simulink model "PannelTest"  (R2022b)
settings: Solver=FixedStepAuto  StartTime=0.0  StopTime=102  FixedStep=0.001  RelTol=1e-3
model workspace (MAT data in the model file):
  Manual_Auto : Simulink.Parameter (value not decoded)
  Pattern : Simulink.Parameter (value not decoded)
  Pause_Start : Simulink.Parameter (value not decoded)
  Stop : Simulink.Parameter (value not decoded)
  Unlock_Lock : Simulink.Parameter (value not decoded)
undefined symbols (not defined in the file or in its folder): DiscIntNeverNeededParam
(part 3 of 3)

== stateflow chart PannelTest/PanelController/ControlPannelStateMachine ==
  state Pause
    State = "Pause";
    if(Pause_StartButtonPressed==0)
    Pause_StartButtonPressed_temp = 0;
    end
  state Stop
    (history)
    state Stop
      State = "Stop";
    state LowerLimb_Follow
      state LowerLimb_Follow
        if(PatternButtonPressed==0)
        PatternButtonPressed_temp = 0;
        end
        State = "Stop";
        Mode = "Lower_Limb_Follow";
        ManualAuto = "";
      (default) -> Stop.LowerLimb_Follow.LowerLimb_Follow
    state LowerLimb_FlutterKick
      (history)
      state LowerLimb_FlutterKick
        if(PatternButtonPressed==0)
        PatternButtonPressed_temp = 0;
        end
        State = "Stop";
        Mode = "Lower_Limb_FlutterKick";
      state LLFK_Manual_Torque
        if(PatternButtonPressed==0)
        PatternButtonPressed_temp = 0;
        end
        if(Manual_AutoButtonPressed==0)
        Manual_AutoButtonPressed_temp = 0;
        end
        State = "Stop";
        Mode = "Lower_Limb_FlutterKick";
        ManualAuto = "LLFK_Manual_Torque";
      state LLFK_Manual_Freq
        if(PatternButtonPressed==0)
        PatternButtonPressed_temp = 0;
        end
        if(Manual_AutoButtonPressed==0)
        Manual_AutoButtonPressed_temp = 0;
        end
        State = "Stop";
        Mode = "Lower_Limb_FlutterKick";
        ManualAuto = "LLFK_Manual_Freq";
      state LLFK_Manual_Pos
        if(PatternButtonPressed==0)
        PatternButtonPressed_temp = 0;
        end
        if(Manual_AutoButtonPressed==0)
        Manual_AutoButtonPressed_temp = 0;
        end
        State = "Stop";
        Mode = "Lower_Limb_FlutterKick";
        ManualAuto = "LLFK_Manual_Pos";
      state LLFK_Auto
        if(PatternButtonPressed==0)
        PatternButtonPressed_temp = 0;
        end
        if(Manual_AutoButtonPressed==0)
        Manual_AutoButtonPressed_temp = 0;
        end
        State = "Stop";
        Mode = "Lower_Limb_FlutterKick";
        ManualAuto = "LLFK_Auto";
      (default) -> Stop.LowerLimb_FlutterKick.LowerLimb_FlutterKick
      Stop.LowerLimb_FlutterKick.LowerLimb_FlutterKick -> LLFK_Manual_Freq
      LLFK_Manual_Freq -> LLFK_Manual_Torque : [(Manual_AutoButtonPressed_temp==0)&&(Manual_AutoButtonPressed>0)]{Manual_AutoButtonPressed_temp=1;}
      LLFK_Manual_Torque -> LLFK_Manual_Pos : [(Manual_AutoButtonPressed_temp==0)&&(Manual_AutoButtonPressed>0)]{Manual_AutoButtonPressed_temp=1;}
      LLFK_Auto -> LLFK_Manual_Freq : [(Manual_AutoButtonPressed_temp==0)&&(Manual_AutoButtonPressed>0)]{Manual_AutoButtonPressed_temp=1;}
      LLFK_Manual_Pos -> LLFK_Auto : [(Manual_AutoButtonPressed_temp==0)&&(Manual_AutoButtonPressed>0)]{Manual_AutoButtonPressed_temp=1;}
    state LowerLimb_Breaststroke
      (history)
      state Lower_Limb_Breaststroke
        if(PatternButtonPressed==0)
        PatternButtonPressed_temp = 0;
        end
        State = "Stop";
        Mode = "Lower_Limb_Breaststroke";
      state LLB_Manual_Torque
        if(PatternButtonPressed==0)
        PatternButtonPressed_temp = 0;
        end
        if(Manual_AutoButtonPressed==0)
        Manual_AutoButtonPressed_temp = 0;
        end
        State = "Stop";
        Mode = "Lower_Limb_Breaststroke";
        ManualAuto = "LLB_Manual_Torque";
      state LLB_Manual_Freq
        if(PatternButtonPressed==0)
        PatternButtonPressed_temp = 0;
        end
        if(Manual_AutoButtonPressed==0)
        Manual_AutoButtonPressed_temp = 0;
        end
        State = "Stop";
        Mode = "Lower_Limb_Breaststroke";
        ManualAuto = "LLB_Manual_Freq";
      state LLB_Manual_Pos
        if(PatternButtonPressed==0)
        PatternButtonPressed_temp = 0;
        end
        if(Manual_AutoButtonPressed==0)
        Manual_AutoButtonPressed_temp = 0;
        end
        State = "Stop";
        Mode = "Lower_Limb_Breaststroke";
        ManualAuto = "LLB_Manual_Pos";
      state LLB_Auto
        if(PatternButtonPressed==0)
        PatternButtonPressed_temp = 0;
        end
        if(Manual_AutoButtonPressed==0)
        Manual_AutoButtonPressed_temp = 0;
        end
        State = "Stop";
        Mode = "Lower_Limb_Breaststroke";
        ManualAuto = "LLB_Auto";
      (default) -> Lower_Limb_Breaststroke
      Lower_Limb_Breaststroke -> LLB_Manual_Freq
      LLB_Manual_Freq -> LLB_Manual_Torque : [(Manual_AutoButtonPressed_temp==0)&&(Manual_AutoButtonPressed>0)]{Manual_AutoButtonPressed_temp=1;}
      LLB_Manual_Torque -> LLB_Manual_Pos : [(Manual_AutoButtonPressed_temp==0)&&(Manual_AutoButtonPressed>0)]{Manual_AutoButtonPressed_temp=1;}
      LLB_Auto -> LLB_Manual_Freq : [(Manual_AutoButtonPressed_temp==0)&&(Manual_AutoButtonPressed>0)]{Manual_AutoButtonPressed_temp=1;}
      LLB_Manual_Pos -> LLB_Auto : [(Manual_AutoButtonPressed_temp==0)&&(Manual_AutoButtonPressed>0)]{Manual_AutoButtonPressed_temp=1;}
    state LowerLimb_Walk
      (history)
      state LowerLimb_Walk
        if(PatternButtonPressed==0)
        PatternButtonPressed_temp = 0;
        end
        State = "Stop";
        Mode = "Lower_Limb_Walk";
      state LLW_Manual_Torque
        if(PatternButtonPressed==0)
        PatternButtonPressed_temp = 0;
        end
        if(Manual_AutoButtonPressed==0)
        Manual_AutoButtonPressed_temp = 0;
        end
        State = "Stop";
        Mode = "Lower_Limb_Walk";
        ManualAuto = "LLW_Manual_Torque";
      state LLW_Manual_Freq
        if(PatternButtonPressed==0)
        PatternButtonPressed_temp = 0;
        end
        if(Manual_AutoButtonPressed==0)
        Manual_AutoButtonPressed_temp = 0;
        end
        State = "Stop";
        Mode = "Lower_Limb_Walk";
        ManualAuto = "LLW_Manual_Freq";
      state LLW_Manual_Pos
        if(PatternButtonPressed==0)
        PatternButtonPressed_temp = 0;
        end
        if(Manual_AutoButtonPressed==0)
        Manual_AutoButtonPressed_temp = 0;
        end
        State = "Stop";
        Mode = "Lower_Limb_Walk";
        ManualAuto = "LLW_Manual_Pos";
      state LLW_Auto
        if(PatternButtonPressed==0)
        PatternButtonPressed_temp = 0;
        end
        if(Manual_AutoButtonPressed==0)
        Manual_AutoButtonPressed_temp = 0;
        end
        State = "Stop";
        Mode = "Lower_Limb_Walk";
        ManualAuto = "LLW_Auto";
      (default) -> Stop.LowerLimb_Walk.LowerLimb_Walk
      Stop.LowerLimb_Walk.LowerLimb_Walk -> LLW_Manual_Freq
      LLW_Manual_Freq -> LLW_Manual_Torque : [(Manual_AutoButtonPressed_temp==0)&&(Manual_AutoButtonPressed>0)]{Manual_AutoButtonPressed_temp=1;}
      LLW_Manual_Torque -> LLW_Manual_Pos : [(Manual_AutoButtonPressed_temp==0)&&(Manual_AutoButtonPressed>0)]{Manual_AutoButtonPressed_temp=1;}
      LLW_Auto -> LLW_Manual_Freq : [(Manual_AutoButtonPressed_temp==0)&&(Manual_AutoButtonPressed>0)]{Manual_AutoButtonPressed_temp=1;}
      LLW_Manual_Pos -> LLW_Auto : [(Manual_AutoButtonPressed_temp==0)&&(Manual_AutoButtonPressed>0)]{Manual_AutoButtonPressed_temp=1;}
    (default) -> Stop.Stop
    Stop.Stop -> Stop.LowerLimb_Follow
    Stop.LowerLimb_Follow -> Stop.LowerLimb_FlutterKick : [(PatternButtonPressed_temp==0)&&(PatternButtonPressed>0)]{PatternButtonPressed_temp=1;}
    LowerLimb_Breaststroke -> Stop.LowerLimb_Walk : [(PatternButtonPressed_temp==0)&&(PatternButtonPressed>0)]{PatternButtonPressed_temp=1;}
    Stop.LowerLimb_FlutterKick -> LowerLimb_Breaststroke : [(PatternButtonPressed_temp==0)&&(PatternButtonPressed>0)]{PatternButtonPressed_temp=1;}
    Stop.LowerLimb_Walk -> Stop.LowerLimb_Follow : [(PatternButtonPressed_temp==0)&&(PatternButtonPressed>0)]{PatternButtonPressed_temp=1;}
  state Start
    state Start
      State = "Start";
      if(Pause_StartButtonPressed==0)
      Pause_StartButtonPressed_temp = 0;
      end
    state UpperLimb_Lock
      if(Pause_StartButtonPressed==0)
      Pause_StartButtonPressed_temp = 0;
      end
      if(Unlock_LockButtonPressed==0)
      Unlock_LockButtonPressed_temp = 0;
      end
      State = "Start";
      UnlockLock = "UpperLimb_Lock";
    state UpperLimb_UnLock
      if(Pause_StartButtonPressed==0)
      Pause_StartButtonPressed_temp = 0;
      end
      if(Unlock_LockButtonPressed==0)
      Unlock_LockButtonPressed_temp = 0;
      end
      State = "Start";
      UnlockLock = "UpperLimb_Unlock";
    (default) -> Start.Start
    Start.Start -> UpperLimb_UnLock
    UpperLimb_Lock -> UpperLimb_UnLock : [(Unlock_LockButtonPressed_temp==0)&&(Unlock_LockButtonPressed>0)]{Unlock_LockButtonPressed_temp=1;}
    UpperLimb_UnLock -> UpperLimb_Lock : [(Unlock_LockButtonPressed_temp==0)&&(Unlock_LockButtonPressed>0)]{Unlock_LockButtonPressed_temp=1;}
  Start -> Pause : [(Pause_StartButtonPressed_temp==0)&&(Pause_StartButtonPressed>0)]{Pause_StartButtonPressed_temp=1;UnlockLock = "UpperLimb_Unlock";}
  Pause -> Stop [order 2] : [StopButtonPressed>0]
  Pause -> Start [order 1] : [(Pause_StartButtonPressed_temp==0)&&(Pause_StartButtonPressed>0)&&(TaskFinished==9)]{Pause_StartButtonPressed_temp=1;}
  (default) -> Stop
  Stop -> Start : [(Pause_StartButtonPressed>0)&&(TaskFinished==1)]{Pause_StartButtonPressed_temp=1;}
  data: TaskFinished input; StopButtonPressed input; State output; Pause_StartButtonPressed input; Pause_StartButtonPressed_temp local; PatternButtonPressed input; Manual_AutoButtonPressed input; Manual_AutoButtonPressed_temp local; PatternButtonPressed_temp local; Mode output string; ManualAuto output string; UnlockLock output string; Unlock_LockButtonPressed input; Unlock_LockButtonPressed_temp local

== stateflow chart PannelTest/PanelController/UpperLimbTaskControlStateMachine ==
  state PauseTask
    ControlState = 1;
  state StopTask
    ControlState = 1;
  state StartTask
    state UnlockTask
      ControlState = 1;
    state LockTask
      ControlState = 2;
    (default) -> UnlockTask
    UnlockTask -> LockTask : [UnlockLock=="UpperLimb_Lock"]
    LockTask -> UnlockTask : [UnlockLock=="UpperLimb_Unlock"]
  (default) -> PauseTask
  PauseTask -> StartTask [order 2] : [State=="Start"]
  PauseTask -> StopTask [order 1] : [State=="Stop"]
  StartTask -> PauseTask : [State=="Pause"]
  StopTask -> StartTask : [State=="Start"]
  data: TaskFinished input; State input; UnlockLock input; ControlState output

== matlab function PannelTest/Tasks/StopTask/MATLAB Function4 ==
  data: u input; y output; Pos input
function y = Current_P(u, Pos)
y = sign(u)*min(abs(u),abs(Pos)*0.1);
